simulink model "dVRK_ToFixedSampleTime_xyz"  (Simulink 8.5)
settings: Solver=ode4  StartTime=0.0  StopTime=length(Tm)/1000  FixedStep=0.001  RelTol=1e-3
settings Model: Creator=HapticLab  LastModifiedBy=HapticLab
settings DataIOCC: SignalLoggingSaveFormat=Dataset
settings OptimizationCC: ExpressionDepthLimit=128
settings DebuggingCC: UnderspecifiedInitializationDetection=Simplified  MergeDetectMultiDrivingBlocksExec=error  FcnCallInpInsideContextMsg=EnableAllAsError  StateNameClashWarn=none
settings GRTTargetCC: CombineOutputUpdateFcns=on  GRTInterface=off

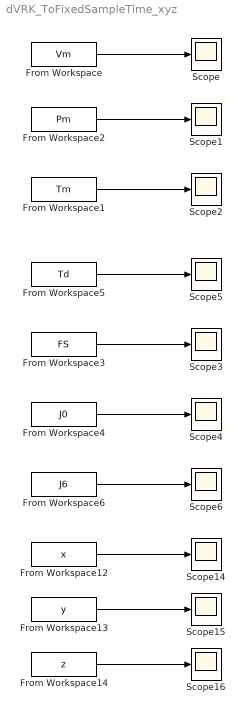
== system dVRK_ToFixedSampleTime_xyz ==
  From Workspace : FromWorkspace  VariableName=Vm  SampleTime=0
  From Workspace1 : FromWorkspace  VariableName=Tm  SampleTime=0
  From Workspace12 : FromWorkspace  VariableName=x  SampleTime=0
  From Workspace13 : FromWorkspace  VariableName=y  SampleTime=0
  From Workspace14 : FromWorkspace  VariableName=z  SampleTime=0
  From Workspace2 : FromWorkspace  VariableName=Pm  SampleTime=0
  From Workspace3 : FromWorkspace  VariableName=FS  SampleTime=0
  From Workspace4 : FromWorkspace  VariableName=J0  SampleTime=0
  From Workspace5 : FromWorkspace  VariableName=Td  SampleTime=0
  From Workspace6 : FromWorkspace  VariableName=J6  SampleTime=0
  Scope{,1..6,14..16} (10 alike) : Scope
      Scope settings: YMin=-2  YMax=3.25  SaveName=Vms
      Scope1 settings: YMin=-3250  YMax=1000  SaveName=Pms
      Scope14 settings: SaveName=Xs
      Scope15 settings: SaveName=Ys
      Scope16 settings: SaveName=Zs
      Scope2 settings: SaveName=Tms
      Scope3 settings: YMin=-11  YMax=7  SaveName=FSs
      Scope4 settings: SaveName=J0s
      Scope5 settings: SaveName=Tds
      Scope6 settings: SaveName=J6s
  wires:
  From Workspace4/1 -> Scope4/1
  From Workspace6/1 -> Scope6/1
  From Workspace5/1 -> Scope5/1
  From Workspace2/1 -> Scope1/1
  From Workspace/1 -> Scope/1
  From Workspace1/1 -> Scope2/1
  From Workspace3/1 -> Scope3/1
  From Workspace12/1 -> Scope14/1
  From Workspace13/1 -> Scope15/1
  From Workspace14/1 -> Scope16/1
